simulink model "freebody_simulation_with_wind"  (R2018b)
settings: Solver=VariableStepAuto  StartTime=0.0  StopTime=40  RelTol=1e-3
undefined symbols (not defined in the file or in its folder): aerosurface_property, GeometryMass
libraries: vrlib x2
settings Model: Creator=lamy  LastModifiedBy=lamy
settings DebuggingCC: LibraryContextMissingDiagnostic=none
settings SFSimCC: SimUseLocalCustomCode=off
settings RTWCC: RTWUseLocalCustomCode=off

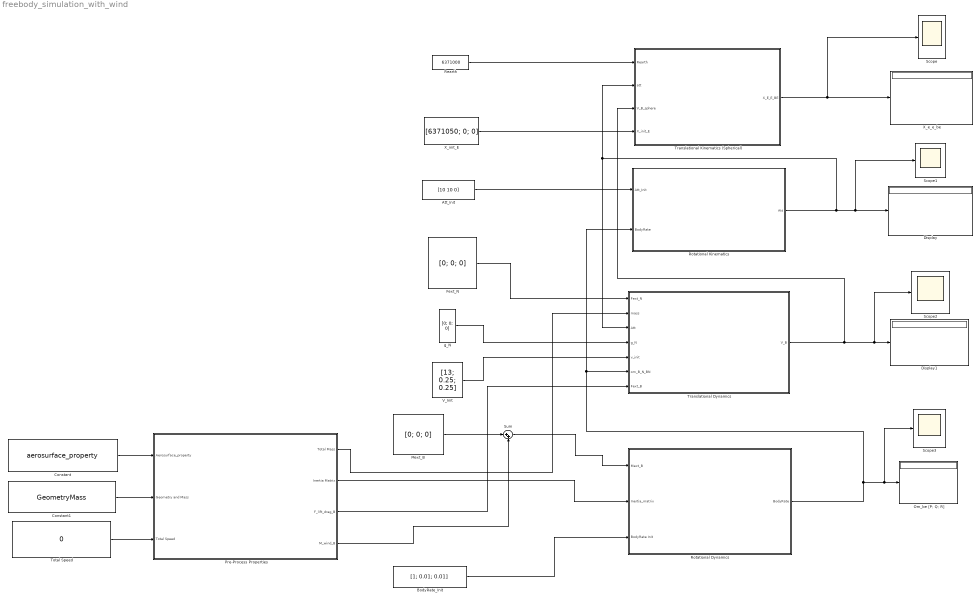
== system freebody_simulation_with_wind ==
  Att_Init : Constant  Value=[10 10 0]
  BodyRate_Init : Constant  Value=[1; 0.01; 0.01]
  Constant : Constant  Value=aerosurface_property  VectorParams1D=off
  Constant1 : Constant  Value=GeometryMass  VectorParams1D=off
  Display : Display
  Display1 : Display
  Fext_N : Constant  Value=[0; 0; 0]  VectorParams1D=off
  Mext_B : Constant  Value=[0; 0; 0]  VectorParams1D=off
  Om_be [P; Q; R] : Display
  Pre-Process Properties : Subsystem
  Rearth : Constant  Value=6371000
  Rotational Dynamics : Subsystem
  Rotational Kinematics : Subsystem
  Scope{,1..3} (4 alike) : Scope
  Sum : Sum  Inputs=|++
  Total Speed : Constant  Value=0  VectorParams1D=off
  Translational Dynamics : Subsystem
  Translational Kinematics (Spherical) : Subsystem
  V_Init : Constant  Value=[13; 0.25; 0.25]  VectorParams1D=off
  X_e_e_be : Display
  X_init_E : Constant  Value=[6371050; 0; 0]
  g_N : Constant  Value=[0; 0; 0]  VectorParams1D=off
  wires:
  Rotational Kinematics/1(Att) -> Scope1/1, Display/1, Translational Kinematics (Spherical)/2(att), Translational Dynamics/3(Att)
  Translational Kinematics (Spherical)/1(X_E_E_BE) -> Scope/1, X_e_e_be/1
  X_init_E/1 -> Translational Kinematics (Spherical)/4(X_init_E)
  BodyRate_Init/1 -> Rotational Dynamics/3(BodyRate Init)
  Rotational Dynamics/1(BodyRate) -> Scope3/1, Om_be [P; Q; R]/1, Translational Dynamics/6(om_B_N_BN), Rotational Kinematics/2(BodyRate)
  Att_Init/1 -> Rotational Kinematics/1(Att_Init)
  V_Init/1 -> Translational Dynamics/5(v_init)
  g_N/1 -> Translational Dynamics/4(g_N)
  Rearth/1 -> Translational Kinematics (Spherical)/1(Rearth)
  Fext_N/1 -> Translational Dynamics/1(Fext_N)
  Constant/1 -> Pre-Process Properties/1(Aerosurface_property)
  Constant1/1 -> Pre-Process Properties/2(Geometry and Mass)
  Total Speed/1 -> Pre-Process Properties/3(Total Speed)
  Pre-Process Properties/1(Total Mass) -> Translational Dynamics/2(mass)
  Pre-Process Properties/2(Inertia Matrix) -> Rotational Dynamics/2(Inertia_matrix)
  Pre-Process Properties/3(F_lift_drag_B) -> Translational Dynamics/7(Fext_B)
  Mext_B/1 -> Sum/1
  Pre-Process Properties/4(M_wind_B) -> Sum/2
  Sum/1 -> Rotational Dynamics/1(Mext_B)
  Translational Dynamics/1(V_B) -> Translational Kinematics (Spherical)/3(V_B_sphere), Scope2/1, Display1/1

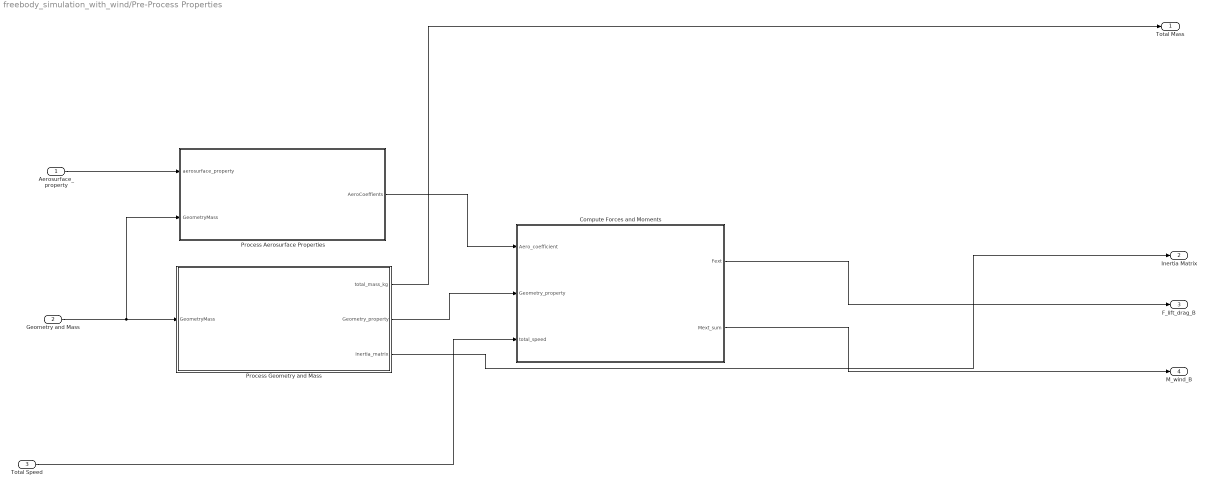
== system freebody_simulation_with_wind/Pre-Process Properties ==
  Aerosurface_property : Inport
  Geometry and Mass : Inport  Port=2
  Total Speed : Inport  Port=3
  Compute Forces and Moments : MATLAB Function  TreatAsAtomicUnit=on
  Process Aerosurface Properties : MATLAB Function  TreatAsAtomicUnit=on
  Process Geometry and Mass : MATLAB Function  TreatAsAtomicUnit=on
  Total Mass : Outport
  Inertia Matrix : Outport  Port=2
  F_lift_drag_B : Outport  Port=3
  M_wind_B : Outport  Port=4
  wires:
  Compute Forces and Moments/2(Mext_sum) -> M_wind_B/1
  Geometry and Mass/1 -> Process Geometry and Mass/1(GeometryMass), Process Aerosurface Properties/2(GeometryMass)
  Compute Forces and Moments/1(Fext) -> F_lift_drag_B/1
  Process Geometry and Mass/1(total_mass_kg) -> Total Mass/1
  Process Aerosurface Properties/1(AeroCoeffients) -> Compute Forces and Moments/1(Aero_coefficient)
  Process Geometry and Mass/2(Geometry_property) -> Compute Forces and Moments/2(Geometry_property)
  Process Geometry and Mass/3(Inertia_matrix) -> Inertia Matrix/1
  Aerosurface_property/1 -> Process Aerosurface Properties/1(aerosurface_property)
  Total Speed/1 -> Compute Forces and Moments/3(total_speed)

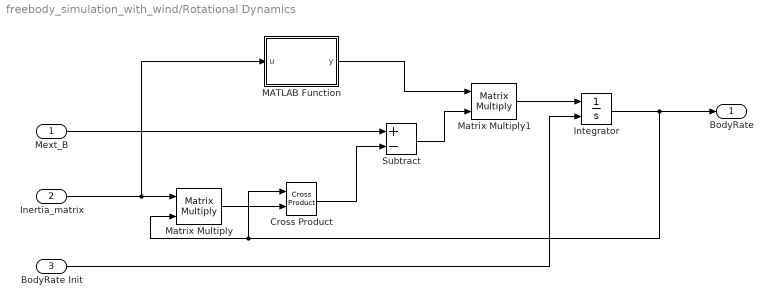
== system freebody_simulation_with_wind/Rotational Dynamics ==
  Mext_B : Inport
  Inertia_matrix : Inport  Port=2
  BodyRate Init : Inport  Port=3
  Cross Product : vrlib/Utilities/Cross Product
      settings: SourceProductBaseCode=VR
  Integrator : Integrator  InitialConditionSource=external
  MATLAB Function : MATLAB Function  TreatAsAtomicUnit=on
  Matrix Multiply : Product  Multiplication=Matrix(*)
  Matrix Multiply1 : Product  Multiplication=Matrix(*)
  Subtract : Sum  Inputs=+-
  BodyRate : Outport
  wires:
  BodyRate Init/1 -> Integrator/2
  Cross Product/1 -> Subtract/2
  Mext_B/1 -> Subtract/1
  MATLAB Function/1(y) -> Matrix Multiply1/1
  Subtract/1 -> Matrix Multiply1/2
  Matrix Multiply1/1 -> Integrator/1
  Matrix Multiply/1 -> Cross Product/2
  Inertia_matrix/1 -> MATLAB Function/1(u), Matrix Multiply/1
  Integrator/1 -> BodyRate/1, Cross Product/1, Matrix Multiply/2

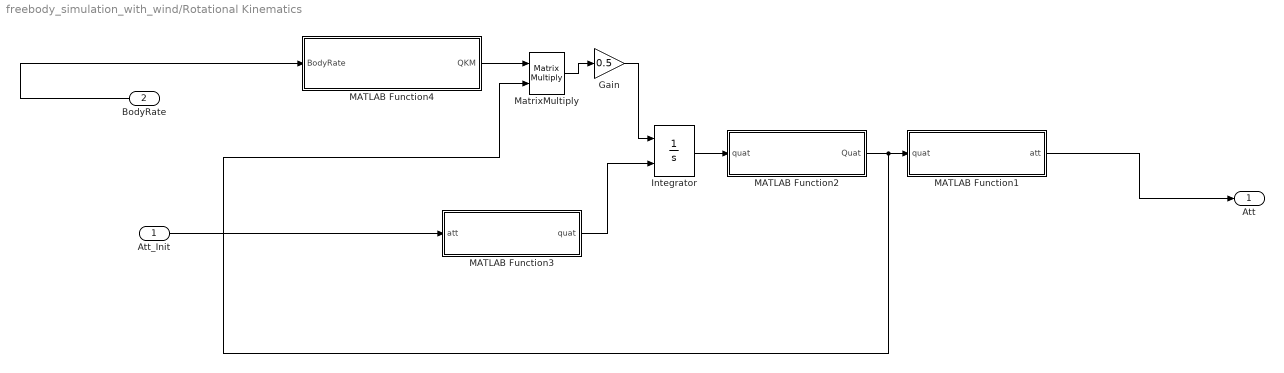
== system freebody_simulation_with_wind/Rotational Kinematics ==
  Att_Init : Inport
  BodyRate : Inport  Port=2
  Gain : Gain  Gain=0.5
  Integrator : Integrator  InitialConditionSource=external
  MATLAB Function1 : MATLAB Function  TreatAsAtomicUnit=on
  MATLAB Function2 : MATLAB Function  TreatAsAtomicUnit=on
  MATLAB Function3 : MATLAB Function  TreatAsAtomicUnit=on
  MATLAB Function4 : MATLAB Function  TreatAsAtomicUnit=on
  MatrixMultiply : Product  Multiplication=Matrix(*)
  Att : Outport
  wires:
  Att_Init/1 -> MATLAB Function3/1(att)
  Integrator/1 -> MATLAB Function2/1(quat)
  MATLAB Function3/1(quat) -> Integrator/2
  Gain/1 -> Integrator/1
  MATLAB Function4/1(QKM) -> MatrixMultiply/1
  MatrixMultiply/1 -> Gain/1
  MATLAB Function2/1(Quat) -> MatrixMultiply/2, MATLAB Function1/1(quat)
  BodyRate/1 -> MATLAB Function4/1(BodyRate)
  MATLAB Function1/1(att) -> Att/1

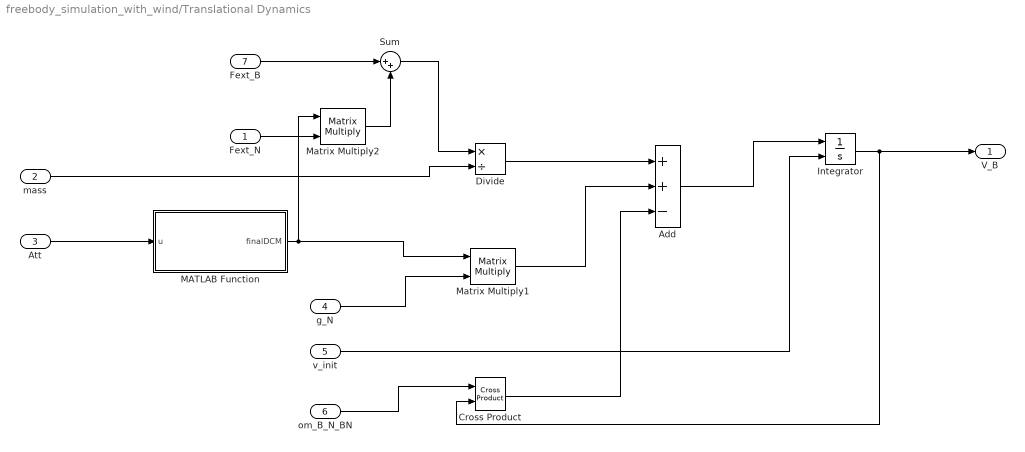
== system freebody_simulation_with_wind/Translational Dynamics ==
  Fext_N : Inport
  mass : Inport  Port=2
  Att : Inport  Port=3
  g_N : Inport  Port=4
  v_init : Inport  Port=5
  om_B_N_BN : Inport  Port=6
  Fext_B : Inport  Port=7
  Add : Sum  Inputs=++-
  Cross Product : vrlib/Utilities/Cross Product
      settings: SourceProductBaseCode=VR
  Divide : Product  Inputs=*/
  Integrator : Integrator  InitialConditionSource=external
  MATLAB Function : MATLAB Function  TreatAsAtomicUnit=on
  Matrix Multiply1 : Product  Multiplication=Matrix(*)
  Matrix Multiply2 : Product  Multiplication=Matrix(*)
  Sum : Sum  Inputs=|++
  V_B : Outport
  wires:
  Matrix Multiply1/1 -> Add/2
  Cross Product/1 -> Add/3
  om_B_N_BN/1 -> Cross Product/1
  Divide/1 -> Add/1
  Att/1 -> MATLAB Function/1(u)
  Integrator/1 -> V_B/1, Cross Product/2
  mass/1 -> Divide/2
  Add/1 -> Integrator/1
  g_N/1 -> Matrix Multiply1/2
  v_init/1 -> Integrator/2
  Fext_N/1 -> Matrix Multiply2/2
  MATLAB Function/1(finalDCM) -> Matrix Multiply1/1, Matrix Multiply2/1
  Fext_B/1 -> Sum/1
  Matrix Multiply2/1 -> Sum/2
  Sum/1 -> Divide/1

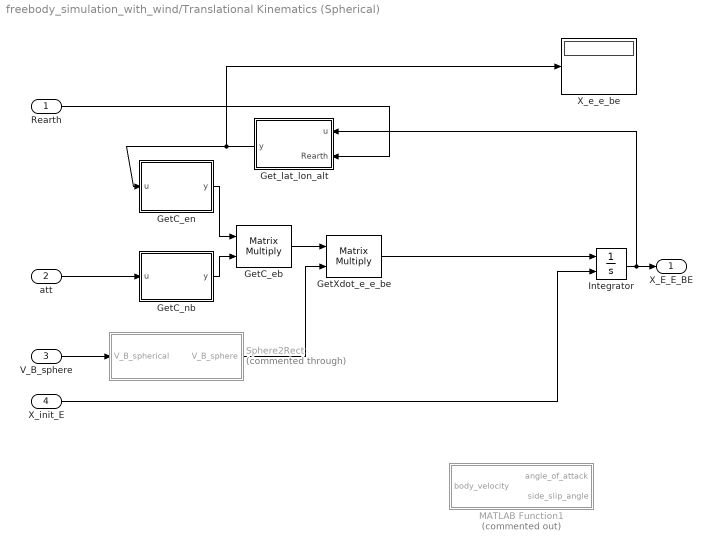
== system freebody_simulation_with_wind/Translational Kinematics (Spherical) ==
  Rearth : Inport
  att : Inport  Port=2
  V_B_sphere : Inport  Port=3
  X_init_E : Inport  Port=4
  GetC_eb : Product  Multiplication=Matrix(*)
  GetC_en : MATLAB Function  TreatAsAtomicUnit=on
  GetC_nb : MATLAB Function  TreatAsAtomicUnit=on
  GetXdot_e_e_be : Product  Multiplication=Matrix(*)
  "Get_lat_lon_alt " : MATLAB Function  TreatAsAtomicUnit=on
  Integrator : Integrator  InitialConditionSource=external
  MATLAB Function1 : MATLAB Function  Commented=on  TreatAsAtomicUnit=on
  Sphere2Rect : MATLAB Function  Commented=through  TreatAsAtomicUnit=on
  X_e_e_be : Display
  X_E_E_BE : Outport
  wires:
  GetC_nb/1(y) -> GetC_eb/2
  GetC_en/1(y) -> GetC_eb/1
  Integrator/1 -> X_E_E_BE/1, "Get_lat_lon_alt "/1(u)
  Rearth/1 -> "Get_lat_lon_alt "/2(Rearth)
  GetXdot_e_e_be/1 -> Integrator/1
  "Get_lat_lon_alt "/1(y) -> X_e_e_be/1, GetC_en/1(u)
  att/1 -> GetC_nb/1(u)
  GetC_eb/1 -> GetXdot_e_e_be/1
  X_init_E/1 -> Integrator/2
  V_B_sphere/1 -> Sphere2Rect/1(V_B_spherical)
  Sphere2Rect/1(V_B_sphere) -> GetXdot_e_e_be/2

== matlab function freebody_simulation_with_wind/Rotational Kinematics/MATLAB Function1 ==
  data: quat input; att output
function att = quat2att(quat)
yaw = atan2(2*(quat(1)*quat(4) + quat(2)*quat(3)), 1-2*(quat(3)^2 + quat(4)^2));
pitch = asin(2*(quat(1)*quat(3) - quat(2)*quat(4)));
roll = atan2(2*(quat(1)*quat(2) + quat(3)*quat(4)), 1-2*(quat(2)^2 + quat(3)^2));
att = [roll; pitch; yaw];

== matlab function freebody_simulation_with_wind/Rotational Kinematics/MATLAB Function4 ==
  data: BodyRate input; QKM output
function QKM = RotKin(BodyRate)
p=BodyRate(1);
q=BodyRate(2);
r=BodyRate(3);
QKM=[ 0,-p,-q,-r;
p, 0, r,-q;
q,-r, 0, p;
r, q,-p, 0];
%q = 0.5*(QKM*quat);

== matlab function freebody_simulation_with_wind/Rotational Kinematics/MATLAB Function2 ==
  data: quat input; Quat output
function Quat = quat_normalize(quat)
norm = dot(quat,quat);
Quat = quat/norm;

== matlab function freebody_simulation_with_wind/Rotational Kinematics/MATLAB Function3 ==
  data: att input; quat output
function quat = att2quat(att)
quat = [0;0;0;0];
quat(1) = cos(att(1)/2)*cos(att(2)/2)*cos(att(3)/2) + sin(att(1)/2)*sin(att(2)/2)*sin(att(3)/2);
quat(2) = sin(att(1)/2)*cos(att(2)/2)*cos(att(3)/2) - cos(att(1)/2)*sin(att(2)/2)*sin(att(3)/2);
quat(3) = cos(att(1)/2)*sin(att(2)/2)*cos(att(3)/2) + sin(att(1)/2)*cos(att(2)/2)*sin(att(3)/2);
quat(4) = cos(att(1)/2)*cos(att(2)/2)*sin(att(3)/2) - sin(att(1)/2)*sin(att(2)/2)*cos(att(3)/2);

== matlab function freebody_simulation_with_wind/Translational Dynamics/MATLAB Function ==
  data: u input; finalDCM output
function finalDCM = att2dcm(u)
yawDCM = [ cos(u(3)) sin(u(3)) 0 ;
-sin(u(3)) cos(u(3)) 0 ;
0 0 1 ];
pitchDCM = [ cos(u(2)) 0 -sin(u(2));
0 1 0 ;
sin(u(2)) 0 cos(u(2)) ];
rollDCM = [ 1 0 0 ;
0 cos(u(1)) sin(u(1));
0 -sin(u(1)) cos(u(1)) ];
finalDCM = rollDCM * pitchDCM * yawDCM;

== matlab function freebody_simulation_with_wind/Translational Kinematics (Spherical)/Sphere2Rect ==
  data: V_B_spherical input; V_B_sphere output
function V_B_sphere = Sphere2Rect(V_B_spherical)
alpha = angle_of_attack;
beta = side_slip_angle;
total_speed =100;
V_B_sphere = [total_speed*cos(alpha)*cos(beta);
    total_speed*sin(beta);
    total_speed*sin(alpha)*cos(beta)];
end

== matlab function freebody_simulation_with_wind/Translational Kinematics (Spherical)/GetC_en ==
  data: u input; y output
function y = fcn(u)

C_00  = [ 0         0         1        ;
          0         1         0        ;
         -1         0         0        ];
     
C_lon = [ 1         0         0        ;
          0         cos(u(2)) sin(u(2));
          0        -sin(u(2)) cos(u(2))];
               
C_lat = [ cos(u(1)) 0         sin(u(1));
          0         1         0        ;
         -sin(u(1)) 0         cos(u(1))];
         
   
C_ne = C_lat * C_lon * C_00;
y = C_ne';

== matlab function freebody_simulation_with_wind/Translational Kinematics (Spherical)/GetC_nb ==
  data: u input; y output
function y = fcn(u)

yawDCM   = [ cos(u(3)) sin(u(3)) 0        ;
            -sin(u(3)) cos(u(3)) 0        ;
             0         0         1        ];
         
pitchDCM = [ cos(u(2)) 0        -sin(u(2));
             0         1         0        ;
             sin(u(2)) 0         cos(u(2))];
         
rollDCM  = [ 1         0         0        ;
             0         cos(u(1)) sin(u(1));
             0        -sin(u(1)) cos(u(1))];
         
finalDCM = rollDCM * pitchDCM * yawDCM;
y = finalDCM';

== matlab function freebody_simulation_with_wind/Translational Kinematics (Spherical)/Get_lat_lon_alt  ==
  data: u input; y output; Rearth input
function y = fcn(u, Rearth)

L = sqrt(u(1)^2+u(2)^2+u(3)^2);

lat = asin(u(3)/L);
lon = atan2(u(2),u(1));
alt = L - Rearth;

y = [lat; lon; alt];

== matlab function freebody_simulation_with_wind/Pre-Process Properties/Process Geometry and Mass ==
  data: GeometryMass input; total_mass_kg output; Geometry_property output; Inertia_matrix output
function [total_mass_kg,Geometry_property,Inertia_matrix] = Process_GeoMass(GeometryMass)
[component_count,null] = size(GeometryMass);
total_mass = sum(GeometryMass(:,1)); %in grams
center_of_gravity_local = zeros(component_count,3);
center_of_gravity_global_sum = zeros(1,3);
for i=[1:1:component_count]
    center_of_gravity_global_sum = GeometryMass(i,1).*GeometryMass(i,5:7)+center_of_gravity_global_sum;
    center_of_gravity_local(i,:) = GeometryMass(i,5:7);
end
center_of_gravity_global = center_of_gravity_global_sum./total_mass;
% Inertia_matrix = [1 0 0; 0 1 0; 0 0 1];
J_xx_local = zeros(component_count,1);
J_yy_local = zeros(component_count,1);
J_zz_local = zeros(component_count,1);

for i = [1:1:component_count]
    J_xx_local(i) = 1/12*GeometryMass(i,1)*(GeometryMass(i,3)^2+GeometryMass(i,4)^2)+GeometryMass(i,1)*(center_of_gravity_local(i,1)-center_of_gravity_global(1))^2;
    J_yy_local(i) = 1/12*GeometryMass(i,1)*(GeometryMass(i,2)^2+GeometryMass(i,4)^2)+GeometryMass(i,1)*(center_of_gravity_local(i,2)-center_of_gravity_global(2))^2;
    J_zz_local(i) = 1/12*GeometryMass(i,1)*(GeometryMass(i,2)^2+GeometryMass(i,3)^2)+GeometryMass(i,1)*(center_of_gravity_local(i,3)-center_of_gravity_global(3))^2;
end
J_xx = sum(J_xx_local);
J_yy = sum(J_yy_local);
J_zz = sum(J_zz_local);
Inertia_matrix = [J_xx 0 0;
                    0 J_yy 0;
                    0 0 J_zz];
chord = [GeometryMass(1,2)+GeometryMass(2,2),
    GeometryMass(3,2),
    GeometryMass(5,2),
    GeometryMass(1,2),
    GeometryMass(2,2)];
span = [GeometryMass(1,3),
    GeometryMass(3,3),
    GeometryMass(5,3),
    GeometryMass(1,3),
    GeometryMass(2,3)];
Geometry_property = [chord';span'];
total_mass_kg = total_mass/1000;
end

== matlab function freebody_simulation_with_wind/Pre-Process Properties/Process Aerosurface Properties ==
  data: aerosurface_property input; AeroCoeffients output; GeometryMass input
function AeroCoeffients   = Process_Aerosurface(aerosurface_property,GeometryMass)
%% Aerosurface
% aerosurface_property = [n_s;CL0_s;e_s;i_s;CD0_s;CDa_s;a0_s;CM0_s;CMa_s];
surface_count = 5;
density = 1.225; % Air Density Constant

n_s = aerosurface_property(1:3,:);
CL0_s =  aerosurface_property(4,:);
e_s = aerosurface_property(5,:);
i_s = aerosurface_property(6,:);
CD0_s = aerosurface_property(7,:);
CDa_s = aerosurface_property(8,:);
a0_s = aerosurface_property(9,:);
CM0_s = aerosurface_property(10,:);
CMa_s = aerosurface_property(11,:);

chord = [GeometryMass(1,2)+GeometryMass(2,2),
    GeometryMass(3,2),
    GeometryMass(5,2),
    GeometryMass(1,2),
    GeometryMass(2,2)];
span = [GeometryMass(1,3),
    GeometryMass(3,3),
    GeometryMass(5,3),
    GeometryMass(1,3),
    GeometryMass(2,3)];
area = chord.*span;
position_of_aerosurface = zeros(surface_count,1);
a_s = zeros(surface_count,1);
AR_s = zeros(surface_count,1);
CLa_s = zeros(surface_count,1);
CL_s = zeros(surface_count,1);
CD_s = zeros(surface_count,1);
CM_s = zeros(surface_count,1);
for i=[2:1:surface_count]
    a_s(i) = i_s(i);% -asin(
    AR_s(i) = span(i)/chord(i);
    CLa_s(i) = 2*pi*AR_s(i)/(2+AR_s(i));
    CL_s(i) = CL0_s(i) + CLa_s(i)*a_s(i);
    CD_s(i) = CD0_s(i) + CDa_s(i)*(a_s(i)-a0_s(i)) + CL_s(i)^2/(pi*e_s(i)*AR_s(i));
    CM_s(i) = CM0_s(i) + CMa_s(i)*a_s(i);
    position_of_aerosurface(i) = 0.25*chord(i);
end
AeroCoeffients = [a_s';AR_s';CLa_s';CL_s';CD_s';CM_s';position_of_aerosurface'];
end

== matlab function freebody_simulation_with_wind/Pre-Process Properties/Compute Forces and Moments ==
  data: Aero_coefficient input; Fext output; Mext_sum output; Geometry_property input; total_speed input
function [Fext,Mext_sum]  = compute_force_moment(Aero_coefficient, Geometry_property,total_speed)
%% Forces Moments
density = 1.225; % Air Density Constant
[null,surface_count] = size(Aero_coefficient);
CL_s = Aero_coefficient(4,:);
CD_s = Aero_coefficient(5,:);
CM_s = Aero_coefficient(6,:)
chord = Geometry_property(1,:);
span = Geometry_property(2,:);
area = chord.*span;
Lift = zeros(surface_count,1);
Drag = zeros(surface_count,1);
Mext = zeros(surface_count,1);
for i=[1:1:surface_count]
    Lift(i,1) = CL_s(i)*0.5*density*total_speed^2*area(i);
    Drag(i,1) = CD_s(i)*0.5*density*total_speed^2*area(i);
    Mext(i,1) = CM_s(i)*0.5*density*total_speed^2*area(i)*chord(i);
end
Fext = [-sum(Drag);0;-sum(Lift)];
Mext_sum = [0; -sum(Mext); 0]; %
end

== matlab function freebody_simulation_with_wind/Translational Kinematics (Spherical)/MATLAB Function1 ==
  data: body_velocity input; angle_of_attack output; side_slip_angle output
function [angle_of_attack, side_slip_angle] = Rect2Sphere(body_velocity)
nction [angle_of_attack, side_slip_angle] = Rect2Sphere(body_velocity)
total_speed = norm(body_velocity);
angle_of_attack = atan2(body_velocity(3),body_velocity(1));
side_slip_angle = asin(body_velocity(2)/total_speed);
end

== matlab function freebody_simulation_with_wind/Rotational Dynamics/MATLAB Function ==
  data: u input; y output
function y = inverse(u)

y = inv(u);
